simulink model "homingLoopSim"  (R2021a)
settings: Solver=ode4  StartTime=0.0  StopTime=simTime  FixedStep=h  RelTol=1e-3
values from neighbouring files (symbols this model uses):
  buffer = 0.000001    (= 1e-06)    [HomingLoopAdjoint.m]
  HE = deg2rad(-20)    [HomingLoopAdjoint.m]
  impulse = 1    [HomingLoopAdjoint.m]
  N_prime = 4    [HomingLoopAdjoint.m]
  nt = G(3)    [HomingLoopAdjoint.m]
  T = 1    [HomingLoopAdjoint.m]
  Vc = 4000    [HomingLoopAdjoint.m]
  Vm = 3000    [HomingLoopAdjoint.m]
settings Model: Creator=dariusmensah  LastModifiedBy=dariusmensah

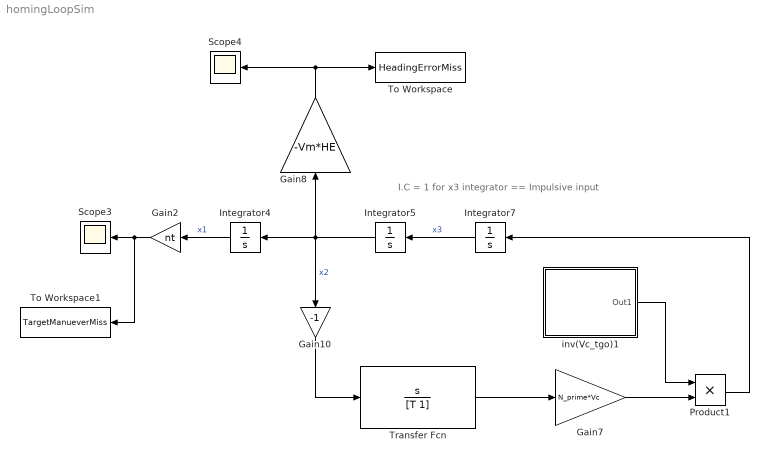
== system homingLoopSim ==
  note: I.C = 1 for x3 integrator == Impulsive input
  Gain10 : Gain  Gain=-1
  Gain2 : Gain  Gain=nt
  Gain7 : Gain  Gain=N_prime*Vc
  Gain8 : Gain  Gain=-Vm*HE
  Integrator4 : Integrator
  Integrator5 : Integrator
  Integrator7 : Integrator  InitialCondition=impulse
  Product1 : Product
  Scope3 : Scope
  Scope4 : Scope
  To Workspace : ToWorkspace  VariableName=HeadingErrorMiss  SaveFormat=Structure With Time  SampleTime=-1
  To Workspace1 : ToWorkspace  VariableName=TargetManueverMiss  SaveFormat=Structure With Time  SampleTime=-1
  Transfer Fcn : TransferFcn  Numerator=[1 0]  Denominator=[T 1]
  inv(Vc_tgo)1 : Subsystem
  wires:
  Gain8/1 -> Scope4/1, To Workspace/1
  Integrator5/1 -> Gain10/1, Integrator4/1, Gain8/1  "x2"
  Product1/1 -> Integrator7/1
  Gain10/1 -> Transfer Fcn/1
  Integrator7/1 -> Integrator5/1  "x3"
  Gain2/1 -> To Workspace1/1, Scope3/1
  Gain7/1 -> Product1/2
  inv(Vc_tgo)1/1(Out1) -> Product1/1
  Integrator4/1 -> Gain2/1  "x1"
  Transfer Fcn/1 -> Gain7/1

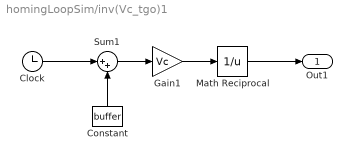
== system homingLoopSim/inv(Vc_tgo)1 ==
  Clock : Clock
  Constant : Constant  Value=buffer
  Gain1 : Gain  Gain=Vc
  Math Reciprocal : Math  Operator=reciprocal  SignedPower=on  SaturateOnIntegerOverflow=on
  Sum1 : Sum  Inputs=|++
  Out1 : Outport
  wires:
  Math Reciprocal/1 -> Out1/1
  Gain1/1 -> Math Reciprocal/1
  Sum1/1 -> Gain1/1
  Constant/1 -> Sum1/2
  Clock/1 -> Sum1/1
